simulink model "controlador_pid"  (R2023b)
settings: Solver=VariableStepAuto  StartTime=0.0  StopTime=10.0  RelTol=1e-3
values from neighbouring files (symbols this model uses):
  ba_num = Jeq_ctrl*n_pid*wn_pid    (= 0.0395694444444)    [controlador_foc_simulink.m]    (also in sistema_completo_en_codigo.m)
  Ksa_num = Jeq_ctrl*n_pid*wn_pid^2    (= 31.6555555556)    [controlador_foc_simulink.m]    (also in sistema_completo_en_codigo.m)
  Ksia_num = Jeq_ctrl*wn_pid^3    (= 10129.7777778)    [controlador_foc_simulink.m]    (also in sistema_completo_en_codigo.m)
settings Model: Creator=Pc  LastModifiedBy=Pc

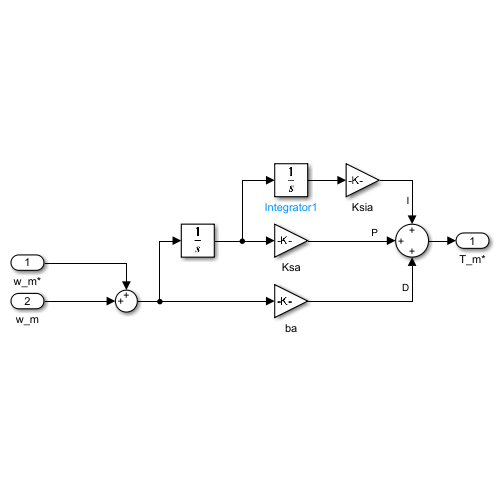
[thumbnail: Simulink's stored preview of the top-level diagram]
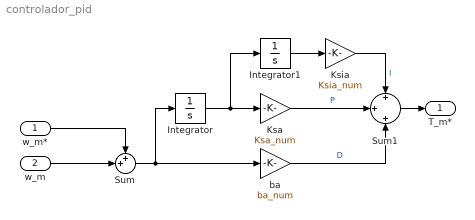
== system controlador_pid ==
  w_m* : Inport
  w_m : Inport  Port=2
  Integrator : Integrator
  Integrator1 : Integrator
  Ksa : Gain  Gain=Ksa_num
  Ksia : Gain  Gain=Ksia_num
  Sum : Sum  Inputs=++|
  Sum1 : Sum  Inputs=+|+|+
  ba : Gain  Gain=ba_num
  T_m* : Outport
  wires:
  w_m*/1 -> Sum/1
  w_m/1 -> Sum/2
  Sum/1 -> Integrator/1, ba/1
  Integrator/1 -> Integrator1/1, Ksa/1
  Integrator1/1 -> Ksia/1
  Sum1/1 -> T_m*/1
  ba/1 -> Sum1/3  "D"
  Ksa/1 -> Sum1/2  "P"
  Ksia/1 -> Sum1/1  "I"
